simulink model "NOx_Aftertratment_Model"  (R2019a)
settings: Solver=VariableStepAuto  StartTime=0.0  StopTime=100  RelTol=1e-3
settings Model: DataDictionary=NOx_Aftertratment_Model_DD.sldd  Creator=Kore  LastModifiedBy=Kore

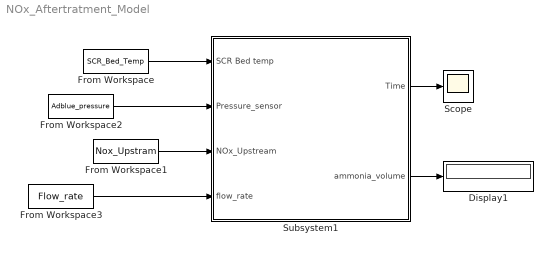
== system NOx_Aftertratment_Model ==
  Display1 : Display
  From Workspace : FromWorkspace  VariableName=SCR_Bed_Temp  SampleTime=0
  From Workspace1 : FromWorkspace  VariableName=Nox_Upstram  SampleTime=0
  From Workspace2 : FromWorkspace  VariableName=Adblue_pressure  SampleTime=0
  From Workspace3 : FromWorkspace  VariableName=Flow_rate  SampleTime=0
  Scope : Scope
  Subsystem1 : Subsystem
  wires:
  From Workspace/1 -> Subsystem1/1(SCR Bed temp)
  From Workspace1/1 -> Subsystem1/3(NOx_Upstream)
  Subsystem1/1(Time) -> Scope/1
  Subsystem1/2(ammonia_volume) -> Display1/1
  From Workspace3/1 -> Subsystem1/4(flow_rate)
  From Workspace2/1 -> Subsystem1/2(Pressure_sensor)

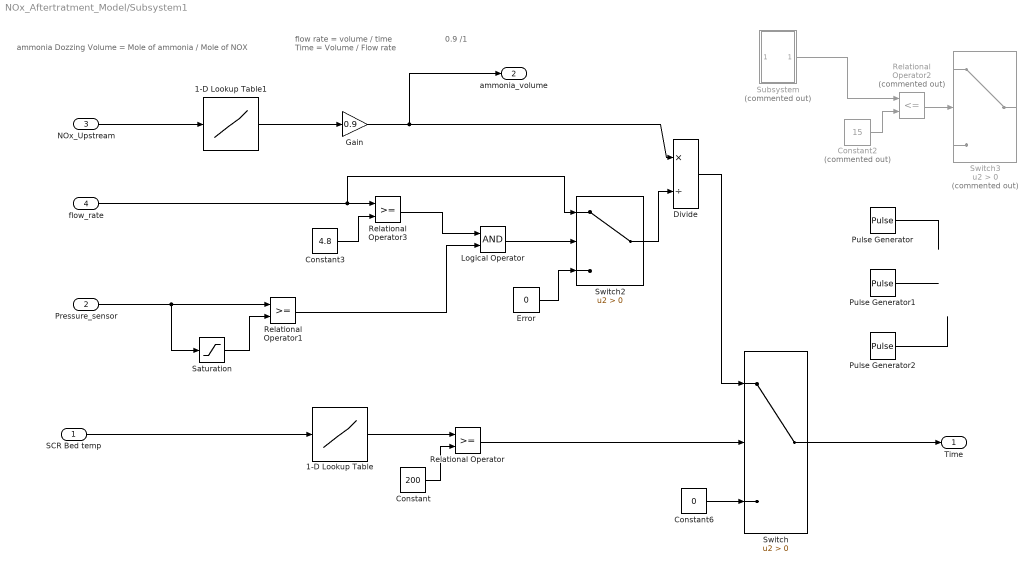
== system NOx_Aftertratment_Model/Subsystem1 ==
  note: 0.9 /1
  note: ammonia Dozzing Volume = Mole of ammonia / Mole of NOX
  note: flow rate = volume / time
      |
      | Time = Volume / Flow rate
  SCR Bed temp : Inport
  Pressure_sensor : Inport  Port=2
  NOx_Upstream : Inport  Port=3
  flow_rate : Inport  Port=4
  1-D Lookup Table : Lookup_n-D  NumberOfTableDimensions=1  BreakpointsForDimension1=[1:10:650]  BreakpointsForDimension2=[1:1:500]  Table=[1:10:650]  InternalRulePriority=Speed  RndMeth=Simplest  InputSameDT=on
  1-D Lookup Table1 : Lookup_n-D  NumberOfTableDimensions=1  BreakpointsForDimension1=[1:5:650]  BreakpointsForDimension2=[1:1:500]  Table=[1:5:650]  InternalRulePriority=Speed  RndMeth=Simplest  InputSameDT=on
  Constant : Constant  Value=200
  Constant2 : Constant  Commented=on  Value=15
  Constant3 : Constant  Value=4.8
  Constant6 : Constant  Value=0
  Divide : Product  Inputs=*/
  Error : Constant  Value=0
  Gain : Gain  Gain=0.9
  Logical Operator : Logic  AllPortsSameDT=off  OutDataTypeStr=boolean
  Pulse Generator : DiscretePulseGenerator  PulseType=Time based  Period=16  PulseWidth=20
  Pulse Generator1 : DiscretePulseGenerator  PulseType=Time based  Period=16  PulseWidth=80
  Pulse Generator2 : DiscretePulseGenerator  PulseType=Time based  Period=16  PulseWidth=60
  Relational Operator : RelationalOperator  OutDataTypeStr=boolean  RndMeth=Simplest
  Relational Operator1 : RelationalOperator  OutDataTypeStr=boolean  RndMeth=Simplest
  Relational Operator2 : RelationalOperator  Commented=on  Operator=<=  OutDataTypeStr=boolean  RndMeth=Simplest
  Relational Operator3 : RelationalOperator  OutDataTypeStr=boolean  RndMeth=Simplest
  Saturation : Saturate  UpperLimit=8  LowerLimit=5
  Subsystem : Subsystem  Commented=on
  Switch : Switch  Criteria=u2 > Threshold
  Switch2 : Switch  Criteria=u2 > Threshold
  Switch3 : Switch  Commented=on  Criteria=u2 > Threshold
  Time : Outport
  ammonia_volume : Outport  Port=2
  wires:
  Constant/1 -> Relational Operator/2
  Saturation/1 -> Relational Operator1/2
  Relational Operator/1 -> Switch/2
  SCR Bed temp/1 -> 1-D Lookup Table/1
  Pressure_sensor/1 -> Saturation/1, Relational Operator1/1
  1-D Lookup Table/1 -> Relational Operator/1
  Constant2/1 -> Relational Operator2/2
  Divide/1 -> Switch/1
  Constant6/1 -> Switch/3
  Relational Operator2/1 -> Switch3/2
  flow_rate/1 -> Switch2/1, Relational Operator3/1
  NOx_Upstream/1 -> 1-D Lookup Table1/1
  Switch2/1 -> Divide/2
  Gain/1 -> ammonia_volume/1, Divide/1
  1-D Lookup Table1/1 -> Gain/1
  Constant3/1 -> Relational Operator3/2
  Error/1 -> Switch2/3
  Switch/1 -> Time/1
  Relational Operator3/1 -> Logical Operator/1
  Relational Operator1/1 -> Logical Operator/2
  Logical Operator/1 -> Switch2/2
  Subsystem/1(Out1) -> Relational Operator2/1
  Pulse Generator/1 -> ?
  Pulse Generator1/1 -> ?
  Pulse Generator2/1 -> ?

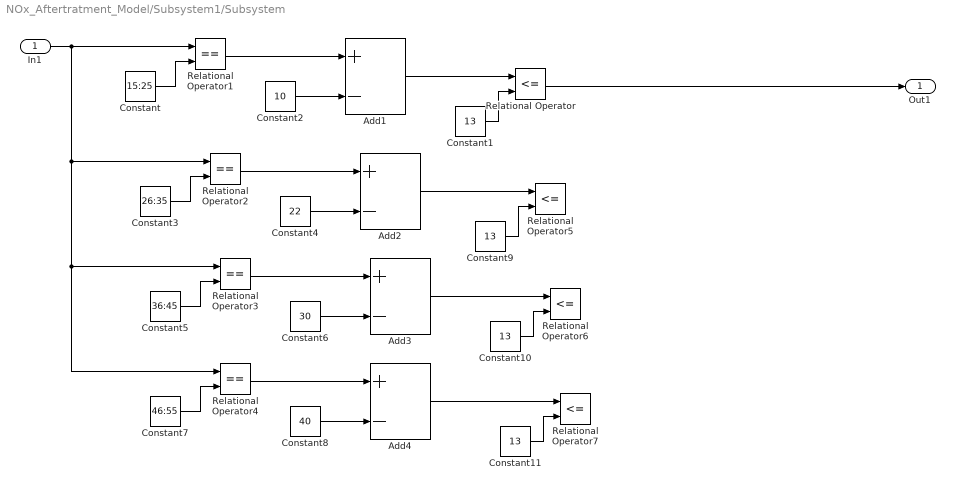
== system NOx_Aftertratment_Model/Subsystem1/Subsystem ==
  In1 : Inport
  Add{1..4} (4 alike) : Sum  Inputs=+-
  Constant : Constant  Value=15:25
  Constant{1,9..11} (4 alike) : Constant  Value=13
  Constant2 : Constant  Value=10
  Constant3 : Constant  Value=26:35
  Constant4 : Constant  Value=22
  Constant5 : Constant  Value=36:45
  Constant6 : Constant  Value=30
  Constant7 : Constant  Value=46:55
  Constant8 : Constant  Value=40
  Relational Operator{,5..7} (4 alike) : RelationalOperator  Operator=<=  OutDataTypeStr=boolean  RndMeth=Simplest
  Relational Operator{1..4} (4 alike) : RelationalOperator  Operator===  OutDataTypeStr=boolean  RndMeth=Simplest
  Out1 : Outport
  wires:
  Add1/1 -> Relational Operator/1
  Constant1/1 -> Relational Operator/2
  Constant/1 -> Relational Operator1/2
  Relational Operator1/1 -> Add1/1
  Constant2/1 -> Add1/2
  Constant4/1 -> Add2/2
  Relational Operator2/1 -> Add2/1
  Constant3/1 -> Relational Operator2/2
  In1/1 -> Relational Operator2/1, Relational Operator3/1, Relational Operator4/1, Relational Operator1/1
  Constant5/1 -> Relational Operator3/2
  Relational Operator3/1 -> Add3/1
  Constant6/1 -> Add3/2
  Constant8/1 -> Add4/2
  Relational Operator4/1 -> Add4/1
  Constant7/1 -> Relational Operator4/2
  Constant9/1 -> Relational Operator5/2
  Add2/1 -> Relational Operator5/1
  Add3/1 -> Relational Operator6/1
  Constant10/1 -> Relational Operator6/2
  Constant11/1 -> Relational Operator7/2
  Add4/1 -> Relational Operator7/1
  Relational Operator/1 -> Out1/1
